simulink model "platform_B3"  (R2019a)
settings: Solver=ode4  StartTime=0.0  StopTime=time_end  FixedStep=Ts  RelTol=1e-3  EnableMultiTasking=on
values from neighbouring files (symbols this model uses):
  taod = 1    [main.m]    (also in plot_M2_SAFETYRADIUS.m; plot_M2_SAFETYRADIUS1.m; plot_M2_SAFETYRADIUS2.m = 2)
  UavTeam = UAVInitialization(M,rm)    [main.m]
settings Model: Creator=Furao  LastModifiedBy=Furao
settings DataIOCC: LimitDataPoints=on  SaveFormat=Array  ReturnWorkspaceOutputs=off  SignalLoggingName=sigsOut
settings DebuggingCC: SaveWithParameterizedLinksMsg=none  UnderspecifiedInitializationDetection=Classic  MergeDetectMultiDrivingBlocksExec=none  SignalResolutionControl=TryResolveAllWithWarning  MultiTaskDSMMsg=warning  MultiTaskCondExecSysMsg=none  ArithmeticOperatorsInVariantConditions=warning
settings HardwareCC: ProdBitPerPointer=32  ProdBitPerSizeT=32  ProdBitPerPtrDiffT=32  ProdLargestAtomicFloat=None  ProdIntDivRoundTo=Undefined  ProdEndianess=Unspecified  ProdWordSize=32  ProdHWDeviceType=32-bit Generic  TargetUnknown=on
settings ModelReferenceCC: PropagateSignalLabelsOutOfModel=off
settings SFSimCC: SimUseLocalCustomCode=off
settings RTWCC: RTWUseLocalCustomCode=off
settings CodeAppCC: StateflowObjectComments=on
settings GRTTargetCC: TargetLangStandard=C89/C90 (ANSI)  CombineOutputUpdateFcns=off  GRTInterface=on
settings ConfigComp: CovMetricSettings=dw  CovHtmlReporting=on  CovSaveCumulativeToWorkspaceVar=on  CovSaveSingleToWorkspaceVar=on  CovExternalEMLEnable=off

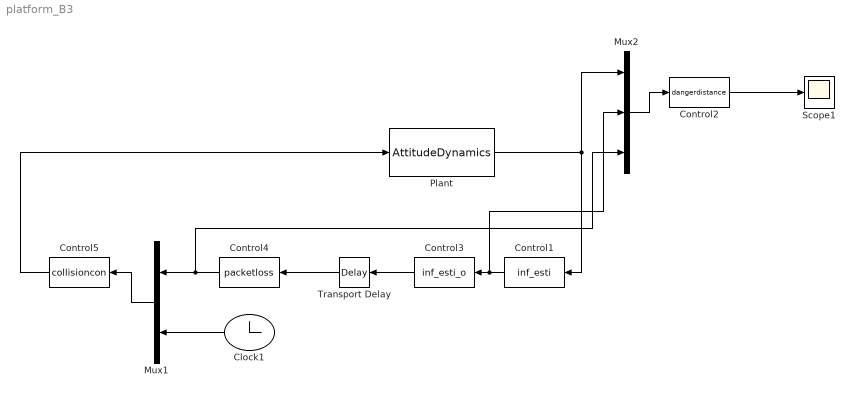
== system platform_B3 ==
  Clock1 : Clock
  Control1 : MATLABFcn  MATLABFcn=inf_esti
  Control2 : MATLABFcn  MATLABFcn=dangerdistance
  Control3 : MATLABFcn  MATLABFcn=inf_esti_o
  Control4 : MATLABFcn  MATLABFcn=packetloss
  Control5 : MATLABFcn  MATLABFcn=collisioncon
  Mux1 : Mux  Inputs=2
  Mux2 : Mux  Inputs=3
  Plant : S-Function  FunctionName=AttitudeDynamics  SFunctionDeploymentMode=off  EnableBusSupport=off
  Scope1 : Scope
  Transport Delay : TransportDelay  DelayTime=taod  InitialOutput=UavTeam.AllHomePos  BufferSize=4096
  wires:
  Plant/1 -> Mux2/1, Control1/1
  Control2/1 -> Scope1/1
  Transport Delay/1 -> Control4/1
  Control4/1 -> Mux2/3, Mux1/1
  Control5/1 -> Plant/1
  Clock1/1 -> Mux1/2
  Mux1/1 -> Control5/1
  Control1/1 -> Mux2/2, Control3/1
  Control3/1 -> Transport Delay/1
  Mux2/1 -> Control2/1
